simulink model "euler321_I2B_12B_with_contracts_EUL001_PP"  (R2017b)
settings: Solver=FixedStepDiscrete  StartTime=0.0  StopTime=10.0  FixedStep=0.010000  RelTol=1e-3  EnableMultiTasking=on
model workspace (MAT data in the model file):
  ContractValidatorBlocksMap = containers.Map
  ContractValidatorBlocksMap.serialization.keys = {'euler321_I2B_12B_with_contracts/euler321_I2B_12B_euler321_Spec/validator', 'euler321_I2B_12B_with_contracts_EUL001/euler321_I2B_12B_euler321_Spec/validator'}
  ContractValidatorBlocksMap.serialization.values{1}.block = 'euler321_I2B_12B_with_contracts/euler321_I2B_12B_euler321_Spec/validator'
  ContractValidatorBlocksMap.serialization.values{1}.assumePorts = 0
  ContractValidatorBlocksMap.serialization.values{1}.guaranteePorts = 9
  ContractValidatorBlocksMap.serialization.values{1}.modeBlocksPorts = 0
  ContractValidatorBlocksMap.serialization.values{1}.portHandles.Inport = [1936.00256348 1938.00256348 1940.00256348 1942.00256348 1944.00256348 1946.00256348 1948.00158691 1950.00256348 1952.00256348]
  ContractValidatorBlocksMap.serialization.values{1}.portHandles.Outport = 2039.00244141
  ContractValidatorBlocksMap.serialization.values{1}.portHandles.Enable = []
  ContractValidatorBlocksMap.serialization.values{1}.portHandles.Trigger = []
  ContractValidatorBlocksMap.serialization.values{1}.portHandles.State = []
  ContractValidatorBlocksMap.serialization.values{1}.portHandles.LConn = []
  ContractValidatorBlocksMap.serialization.values{1}.portHandles.RConn = []
  ContractValidatorBlocksMap.serialization.values{1}.portHandles.Ifaction = []
  ContractValidatorBlocksMap.serialization.values{1}.portHandles.Reset = []
  ContractValidatorBlocksMap.serialization.values{1}.portConnectivity(1).Type = '1'
  ContractValidatorBlocksMap.serialization.values{1}.portConnectivity(1).Position = [2610 2845]
  ContractValidatorBlocksMap.serialization.values{1}.portConnectivity(1).SrcBlock = 1300.00341797
  ContractValidatorBlocksMap.serialization.values{1}.portConnectivity(1).SrcPort = 0
  ContractValidatorBlocksMap.serialization.values{1}.portConnectivity(1).DstBlock = []
  ContractValidatorBlocksMap.serialization.values{1}.portConnectivity(1).DstPort = []
  ContractValidatorBlocksMap.serialization.values{1}.portConnectivity(2).Type = '2'
  ContractValidatorBlocksMap.serialization.values{1}.portConnectivity(2).Position = [2610 2885]
  ContractValidatorBlocksMap.serialization.values{1}.portConnectivity(2).SrcBlock = 1307.00341797
  ContractValidatorBlocksMap.serialization.values{1}.portConnectivity(2).SrcPort = 0
  ContractValidatorBlocksMap.serialization.values{1}.portConnectivity(2).DstBlock = []
  ContractValidatorBlocksMap.serialization.values{1}.portConnectivity(2).DstPort = []
  ContractValidatorBlocksMap.serialization.values{1}.portConnectivity(3).Type = '3'
  ContractValidatorBlocksMap.serialization.values{1}.portConnectivity(3).Position = [2610 2925]
  ContractValidatorBlocksMap.serialization.values{1}.portConnectivity(3).SrcBlock = 1314.00280762
  ContractValidatorBlocksMap.serialization.values{1}.portConnectivity(3).SrcPort = 0
  ContractValidatorBlocksMap.serialization.values{1}.portConnectivity(3).DstBlock = []
  ContractValidatorBlocksMap.serialization.values{1}.portConnectivity(3).DstPort = []
  ContractValidatorBlocksMap.serialization.values{1}.portConnectivity(4).Type = '4'
  ContractValidatorBlocksMap.serialization.values{1}.portConnectivity(4).Position = [2610 2965]
  ContractValidatorBlocksMap.serialization.values{1}.portConnectivity(4).SrcBlock = 1318.00280762
  ContractValidatorBlocksMap.serialization.values{1}.portConnectivity(4).SrcPort = 0
  ContractValidatorBlocksMap.serialization.values{1}.portConnectivity(4).DstBlock = []
  ContractValidatorBlocksMap.serialization.values{1}.portConnectivity(4).DstPort = []
  ContractValidatorBlocksMap.serialization.values{1}.portConnectivity(5).Type = '5'
  ContractValidatorBlocksMap.serialization.values{1}.portConnectivity(5).Position = [2610 3005]
  ContractValidatorBlocksMap.serialization.values{1}.portConnectivity(5).SrcBlock = 1326.00292969
  ContractValidatorBlocksMap.serialization.values{1}.portConnectivity(5).SrcPort = 0
  ContractValidatorBlocksMap.serialization.values{1}.portConnectivity(5).DstBlock = []
  ContractValidatorBlocksMap.serialization.values{1}.portConnectivity(5).DstPort = []
  ContractValidatorBlocksMap.serialization.values{1}.portConnectivity(6).Type = '6'
  ContractValidatorBlocksMap.serialization.values{1}.portConnectivity(6).Position = [2610 3045]
  ContractValidatorBlocksMap.serialization.values{1}.portConnectivity(6).SrcBlock = 1330.00341797
  ContractValidatorBlocksMap.serialization.values{1}.portConnectivity(6).SrcPort = 0
  ContractValidatorBlocksMap.serialization.values{1}.portConnectivity(6).DstBlock = []
  ContractValidatorBlocksMap.serialization.values{1}.portConnectivity(6).DstPort = []
  ContractValidatorBlocksMap.serialization.values{1}.portConnectivity(7).Type = '7'
  ContractValidatorBlocksMap.serialization.values{1}.portConnectivity(7).Position = [2610 3085]
  ContractValidatorBlocksMap.serialization.values{1}.portConnectivity(7).SrcBlock = 1337.00341797
  ContractValidatorBlocksMap.serialization.values{1}.portConnectivity(7).SrcPort = 0
  ContractValidatorBlocksMap.serialization.values{1}.portConnectivity(7).DstBlock = []
  ContractValidatorBlocksMap.serialization.values{1}.portConnectivity(7).DstPort = []
  ContractValidatorBlocksMap.serialization.values{1}.portConnectivity(8).Type = '8'
  ContractValidatorBlocksMap.serialization.values{1}.portConnectivity(8).Position = [2610 3125]
  ContractValidatorBlocksMap.serialization.values{1}.portConnectivity(8).SrcBlock = 1341.00341797
  ContractValidatorBlocksMap.serialization.values{1}.portConnectivity(8).SrcPort = 0
  ContractValidatorBlocksMap.serialization.values{1}.portConnectivity(8).DstBlock = []
  ContractValidatorBlocksMap.serialization.values{1}.portConnectivity(8).DstPort = []
  ContractValidatorBlocksMap.serialization.values{1}.portConnectivity(9).Type = '9'
  ContractValidatorBlocksMap.serialization.values{1}.portConnectivity(9).Position = [2610 3165]
  ContractValidatorBlocksMap.serialization.values{1}.portConnectivity(9).SrcBlock = 1348.00476074
  ContractValidatorBlocksMap.serialization.values{1}.portConnectivity(9).SrcPort = 0
  ContractValidatorBlocksMap.serialization.values{1}.portConnectivity(9).DstBlock = []
  ContractValidatorBlocksMap.serialization.values{1}.portConnectivity(9).DstPort = []
  ContractValidatorBlocksMap.serialization.values{1}.portConnectivity(10).Type = '1'
  ContractValidatorBlocksMap.serialization.values{1}.portConnectivity(10).Position = [2650 3005]
  ContractValidatorBlocksMap.serialization.values{1}.portConnectivity(10).SrcBlock = []
  ContractValidatorBlocksMap.serialization.values{1}.portConnectivity(10).SrcPort = []
  ContractValidatorBlocksMap.serialization.values{1}.portConnectivity(10).DstBlock = 1447.00341797
  ContractValidatorBlocksMap.serialization.values{1}.portConnectivity(10).DstPort = 0
  ContractValidatorBlocksMap.serialization.values{2}.block = 'euler321_I2B_12B_with_contracts_EUL001/euler321_I2B_12B_euler321_Spec/validator'
  ContractValidatorBlocksMap.serialization.values{2}.assumePorts = 0
  ContractValidatorBlocksMap.serialization.values{2}.guaranteePorts = 9
  ContractValidatorBlocksMap.serialization.values{2}.modeBlocksPorts = 0
  ContractValidatorBlocksMap.serialization.values{2}.portHandles.Inport = [497.151367188 498.151367188 499.150512695 500.149414062 501.150268555 502.149169922 503.149047852 504.149536133 505.150024414]
  ContractValidatorBlocksMap.serialization.values{2}.portHandles.Outport = 506.149047852
  ContractValidatorBlocksMap.serialization.values{2}.portHandles.Enable = []
  ContractValidatorBlocksMap.serialization.values{2}.portHandles.Trigger = []
  ContractValidatorBlocksMap.serialization.values{2}.portHandles.State = []
  ContractValidatorBlocksMap.serialization.values{2}.portHandles.LConn = []
  ContractValidatorBlocksMap.serialization.values{2}.portHandles.RConn = []
  ContractValidatorBlocksMap.serialization.values{2}.portHandles.Ifaction = []
  ContractValidatorBlocksMap.serialization.values{2}.portHandles.Reset = []
  ContractValidatorBlocksMap.serialization.values{2}.portConnectivity(1).Type = '1'
  ContractValidatorBlocksMap.serialization.values{2}.portConnectivity(1).Position = [2610 2845]
  ContractValidatorBlocksMap.serialization.values{2}.portConnectivity(1).SrcBlock = 243.150024414
  ContractValidatorBlocksMap.serialization.values{2}.portConnectivity(1).SrcPort = 0
  ContractValidatorBlocksMap.serialization.values{2}.portConnectivity(1).DstBlock = []
  ContractValidatorBlocksMap.serialization.values{2}.portConnectivity(1).DstPort = []
  ContractValidatorBlocksMap.serialization.values{2}.portConnectivity(2).Type = '2'
  ContractValidatorBlocksMap.serialization.values{2}.portConnectivity(2).Position = [2610 2885]
  ContractValidatorBlocksMap.serialization.values{2}.portConnectivity(2).SrcBlock = 247.150024414
  ContractValidatorBlocksMap.serialization.values{2}.portConnectivity(2).SrcPort = 0
  ContractValidatorBlocksMap.serialization.values{2}.portConnectivity(2).DstBlock = []
  ContractValidatorBlocksMap.serialization.values{2}.portConnectivity(2).DstPort = []
  ContractValidatorBlocksMap.serialization.values{2}.portConnectivity(3).Type = '3'
  ContractValidatorBlocksMap.serialization.values{2}.portConnectivity(3).Position = [2610 2925]
  ContractValidatorBlocksMap.serialization.values{2}.portConnectivity(3).SrcBlock = 251.153320312
  ContractValidatorBlocksMap.serialization.values{2}.portConnectivity(3).SrcPort = 0
  ContractValidatorBlocksMap.serialization.values{2}.portConnectivity(3).DstBlock = []
  ContractValidatorBlocksMap.serialization.values{2}.portConnectivity(3).DstPort = []
  ContractValidatorBlocksMap.serialization.values{2}.portConnectivity(4).Type = '4'
  ContractValidatorBlocksMap.serialization.values{2}.portConnectivity(4).Position = [2610 2965]
  ContractValidatorBlocksMap.serialization.values{2}.portConnectivity(4).SrcBlock = 255.153564453
  ContractValidatorBlocksMap.serialization.values{2}.portConnectivity(4).SrcPort = 0
  ContractValidatorBlocksMap.serialization.values{2}.portConnectivity(4).DstBlock = []
  ContractValidatorBlocksMap.serialization.values{2}.portConnectivity(4).DstPort = []
  ContractValidatorBlocksMap.serialization.values{2}.portConnectivity(5).Type = '5'
  ContractValidatorBlocksMap.serialization.values{2}.portConnectivity(5).Position = [2610 3005]
  ContractValidatorBlocksMap.serialization.values{2}.portConnectivity(5).SrcBlock = 259.148925781
  ContractValidatorBlocksMap.serialization.values{2}.portConnectivity(5).SrcPort = 0
  ContractValidatorBlocksMap.serialization.values{2}.portConnectivity(5).DstBlock = []
  ContractValidatorBlocksMap.serialization.values{2}.portConnectivity(5).DstPort = []
  ContractValidatorBlocksMap.serialization.values{2}.portConnectivity(6).Type = '6'
  ContractValidatorBlocksMap.serialization.values{2}.portConnectivity(6).Position = [2610 3045]
  ContractValidatorBlocksMap.serialization.values{2}.portConnectivity(6).SrcBlock = 263.154296875
  ContractValidatorBlocksMap.serialization.values{2}.portConnectivity(6).SrcPort = 0
  ContractValidatorBlocksMap.serialization.values{2}.portConnectivity(6).DstBlock = []
  ContractValidatorBlocksMap.serialization.values{2}.portConnectivity(6).DstPort = []
  ContractValidatorBlocksMap.serialization.values{2}.portConnectivity(7).Type = '7'
  ContractValidatorBlocksMap.serialization.values{2}.portConnectivity(7).Position = [2610 3085]
  ContractValidatorBlocksMap.serialization.values{2}.portConnectivity(7).SrcBlock = 267.154418945
  ContractValidatorBlocksMap.serialization.values{2}.portConnectivity(7).SrcPort = 0
  ContractValidatorBlocksMap.serialization.values{2}.portConnectivity(7).DstBlock = []
  ContractValidatorBlocksMap.serialization.values{2}.portConnectivity(7).DstPort = []
  ContractValidatorBlocksMap.serialization.values{2}.portConnectivity(8).Type = '8'
  ContractValidatorBlocksMap.serialization.values{2}.portConnectivity(8).Position = [2610 3125]
  ContractValidatorBlocksMap.serialization.values{2}.portConnectivity(8).SrcBlock = 271.148925781
  ContractValidatorBlocksMap.serialization.values{2}.portConnectivity(8).SrcPort = 0
  ContractValidatorBlocksMap.serialization.values{2}.portConnectivity(8).DstBlock = []
  ContractValidatorBlocksMap.serialization.values{2}.portConnectivity(8).DstPort = []
  ContractValidatorBlocksMap.serialization.values{2}.portConnectivity(9).Type = '9'
  ContractValidatorBlocksMap.serialization.values{2}.portConnectivity(9).Position = [2610 3165]
  ContractValidatorBlocksMap.serialization.values{2}.portConnectivity(9).SrcBlock = 275.153442383
  ContractValidatorBlocksMap.serialization.values{2}.portConnectivity(9).SrcPort = 0
  ContractValidatorBlocksMap.serialization.values{2}.portConnectivity(9).DstBlock = []
  ContractValidatorBlocksMap.serialization.values{2}.portConnectivity(9).DstPort = []
  ContractValidatorBlocksMap.serialization.values{2}.portConnectivity(10).Type = '1'
  ContractValidatorBlocksMap.serialization.values{2}.portConnectivity(10).Position = [2650 3005]
  ContractValidatorBlocksMap.serialization.values{2}.portConnectivity(10).SrcBlock = []
  ContractValidatorBlocksMap.serialization.values{2}.portConnectivity(10).SrcPort = []
  ContractValidatorBlocksMap.serialization.values{2}.portConnectivity(10).DstBlock = 342.152099609
  ContractValidatorBlocksMap.serialization.values{2}.portConnectivity(10).DstPort = 0
  ContractValidatorBlocksMap.serialization.uniformity = 0
  ContractValidatorBlocksMap.serialization.keyType = 'char'
  ContractValidatorBlocksMap.serialization.valueType = 'any'
  already_pp = 1
  compositionalMap.analysisNames = {'euler321_I2B_12B_with_contracts_EUL001_PP/COORDINATETRANSFORM_newline_EULER321_newline__lpar_INERTIALTOBODY_rpar_'}
  compositionalMap.compositionalOptions = {{''}}
  compositionalMap.selectedOptions = 1
  maskControlsMap = containers.Map
  maskControlsMap.serialization.keys = {'euler321_I2B_12B_with_contracts_EUL001_PP/euler321_I2B_12B_euler321_Spec/EUL001_1', 'euler321_I2B_12B_with_contracts_EUL001_PP/euler321_I2B_12B_euler321_Spec/EUL001_2', 'euler321_I2B_12B_with_contracts_EUL001_PP/euler321_I2B_12B_euler321_Spec/EUL001_3', 'euler321_I2B_12B_with_contracts_EUL001_PP/euler321_I2B_12B_euler321_Spec/EUL001_4', 'euler321_I2B_12B_with_contracts_EUL001_PP/euler321_I2B_12B_euler321_Spec/EUL001_5', 'euler321_I2B_12B_with_contracts_EUL001_PP/euler321_I2B_12B_euler321_Spec/EUL001_6', 'euler321_I2B_12B_with_contracts_EUL001_PP/euler321_I2B_12B_euler321_Spec/EUL001_7', 'euler321_I2B_12B_with_contracts_EUL001_PP/euler321_I2B_12B_euler321_Spec/EUL001_8', 'euler321_I2B_12B_with_contracts_EUL001_PP/euler321_I2B_12B_euler321_Spec/EUL001_9'}
  maskControlsMap.serialization.values = {{'Display_counter_example_as_signals', 'Display_counter_example_as_tables', 'Display_counter_example_as_HTML_tables', 'Generate_an_outer_model_for_the_counter_example', 'Generate_an_inner_model_for_the_counter_example'}, {'Display_counter_example_as_signals', 'Display_counter_example_as_tables', 'Display_counter_example_as_HTML_tables', 'Generate_an_outer_model_for_the_counter_example', 'Generate_an_inner_model_for_the_counter_example'}, {'Display_counter_example_as_signals', 'Display_counter_example_as_tables', 'Display_counter_example_as_HTML_tables', 'Generate_an_outer_model_for_the_counter_example', 'Generate_an_inner_model_for_the_counter_example'}, {'Display_counter_example_as_signals', 'Display_counter_example_as_tables', 'Display_counter_example_as_HTML_tables', 'Generate_an_outer_model_for_the_counter_example', 'Generate_an_inner_model_for_the_counter_example'}, {'Display_counter_example_as_signals', 'Display_counter_example_as_tables', 'Display_counter_example_as_HTML_tables', 'Generate_an_outer_model_for_the_counter_example', 'Generate_an_inner_model_for_the_counter_example'}, {'Display_counter_example_as_signals', 'Display_counter_example_as_tables', 'Display_counter_example_as_HTML_tables', 'Generate_an_outer_model_for_the_counter_example', 'Generate_an_inner_model_for_the_counter_example'}, {'Display_counter_example_as_signals', 'Display_counter_example_as_tables', 'Display_counter_example_as_HTML_tables', 'Generate_an_outer_model_for_the_counter_example', 'Generate_an_inner_model_for_the_counter_example'}, {'Display_counter_example_as_signals', 'Display_counter_example_as_tables', 'Display_counter_example_as_HTML_tables', 'Generate_an_outer_model_for_the_counter_example', 'Generate_an_inner_model_for_the_counter_example'}, {'Display_counter_example_as_signals', 'Display_counter_example_as_tables', 'Display_counter_example_as_HTML_tables', 'Generate_an_outer_model_for_the_counter_example', 'Generate_an_inner_model_for_the_counter_example'}}
  maskControlsMap.serialization.uniformity = 0
  maskControlsMap.serialization.keyType = 'char'
  maskControlsMap.serialization.valueType = 'any'
  nodeNameToBlockNameMap : containers.Map (value not decoded)
  verificationResults : struct (value not decoded)
undefined symbols (not defined in the file): contractAfterSimulation, contractBeforeSimulation, ContractBlock, ContractGuaranteeBlock, ContractValidatorBlock, saveValidatorParameters
settings Model: Creator=elliocm  LastModifiedBy=hbourbou
settings DataIOCC: LimitDataPoints=on  SaveFormat=StructureWithTime  SignalLoggingSaveFormat=ModelDataLogs
settings OptimizationCC: ExpressionDepthLimit=2147483647  LifeSpan=inf
settings DebuggingCC: AlgebraicLoopMsg=error  ArtificialAlgebraicLoopMsg=error  UnderspecifiedInitializationDetection=Classic  MergeDetectMultiDrivingBlocksExec=none  SolverPrmCheckMsg=warning  SingleTaskRateTransMsg=error  FcnCallInpInsideContextMsg=warning  StateNameClashWarn=warning  SFUnexpectedBacktrackingDiag=warning  SFNoUnconditionalDefaultTransitionDiag=warning  SFExecutionAtInitializationDiag=none
settings HardwareCC: ProdBitPerPointer=32  ProdBitPerSizeT=32  ProdBitPerPtrDiffT=32  ProdLargestAtomicFloat=None  ProdIntDivRoundTo=Undefined  ProdEndianess=Unspecified  ProdWordSize=32  ProdHWDeviceType=32-bit Generic
settings ModelReferenceCC: PropagateSignalLabelsOutOfModel=off
settings CodeAppCC: StateflowObjectComments=on
settings GRTTargetCC: TargetLangStandard=C89/C90 (ANSI)  GeneratePreprocessorConditionals=Disable all  CombineOutputUpdateFcns=off  GRTInterface=on
settings ConfigComp: CovMetricSettings=dw  CovHtmlReporting=on  CovSaveCumulativeToWorkspaceVar=on  CovSaveSingleToWorkspaceVar=on  CovExternalEMLEnable=off

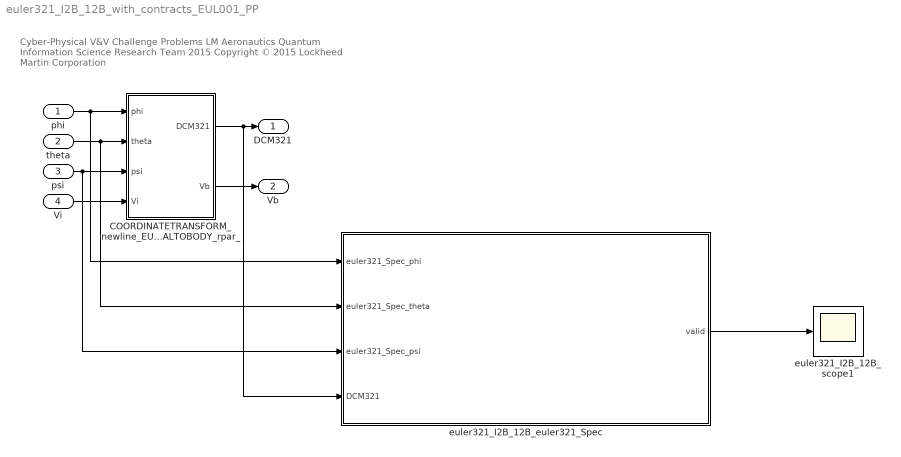
== system euler321_I2B_12B_with_contracts_EUL001_PP ==
  note: Cyber-Physical V&V Challenge Problems
      | LM Aeronautics Quantum Information Science Research Team 2015
      | Copyright © 2015 Lockheed Martin Corporation
  phi : Inport  OutDataTypeStr=double
  theta : Inport  Port=2  OutDataTypeStr=double
  psi : Inport  Port=3  OutDataTypeStr=double
  Vi : Inport  Port=4  OutDataTypeStr=double  PortDimensions=3
  COORDINATETRANSFORM_newline_EULER321_newline__lpar_INERTIALTOBODY_rpar_ : Subsystem  TreatAsAtomicUnit=on
  euler321_I2B_12B_euler321_Spec : Subsystem  TreatAsAtomicUnit=on  mask(ContractBlock){ContractBlockType=ContractBlock}
      mask init:
      | set_param(gcb, 'LinkStatus', 'none');
      mask DialogControl DescTextVar Prompt: Contract block
      mask Display:
      | text(0.5, 0.5, '{\bf\fontsize{20}Contract}', 'hor', 'center', 'texmode','on');
      | blocks = find_system(gcb, 'LookUnderMasks','all', 'SearchDepth',1,'BlockType','Inport');
      | for i = 1 : length(blocks)
      |     blockName = get_param(blocks(i), 'Name');
      |     [path, blockName] = fileparts(char(blockName));
      |     port_label('input', i, blockName);
      | end
      | 
      | blocks = find_system(gcb, 'LookUnderMasks','all', 'SearchDepth',1,'BlockType','Outport');
      | for i = 1 : length(blocks)
      |     blockName = get_param(blocks(i), 'Name');
      |     [path, blockName] = fileparts(char(blockName));
      |     port_label('output', i, blockName);
      | end
  euler321_I2B_12B_scope1 : Scope
  DCM321 : Outport  VectorParamsAs1DForOutWhenUnconnected=off
  Vb : Outport  Port=2  VectorParamsAs1DForOutWhenUnconnected=off
  wires:
  COORDINATETRANSFORM_newline_EULER321_newline__lpar_INERTIALTOBODY_rpar_/1(DCM321) -> euler321_I2B_12B_euler321_Spec/4(DCM321), DCM321/1
  COORDINATETRANSFORM_newline_EULER321_newline__lpar_INERTIALTOBODY_rpar_/2(Vb) -> Vb/1
  phi/1 -> COORDINATETRANSFORM_newline_EULER321_newline__lpar_INERTIALTOBODY_rpar_/1(phi), euler321_I2B_12B_euler321_Spec/1(euler321_Spec_phi)
  theta/1 -> euler321_I2B_12B_euler321_Spec/2(euler321_Spec_theta), COORDINATETRANSFORM_newline_EULER321_newline__lpar_INERTIALTOBODY_rpar_/2(theta)
  psi/1 -> COORDINATETRANSFORM_newline_EULER321_newline__lpar_INERTIALTOBODY_rpar_/3(psi), euler321_I2B_12B_euler321_Spec/3(euler321_Spec_psi)
  Vi/1 -> COORDINATETRANSFORM_newline_EULER321_newline__lpar_INERTIALTOBODY_rpar_/4(Vi)
  euler321_I2B_12B_euler321_Spec/1(valid) -> euler321_I2B_12B_scope1/1

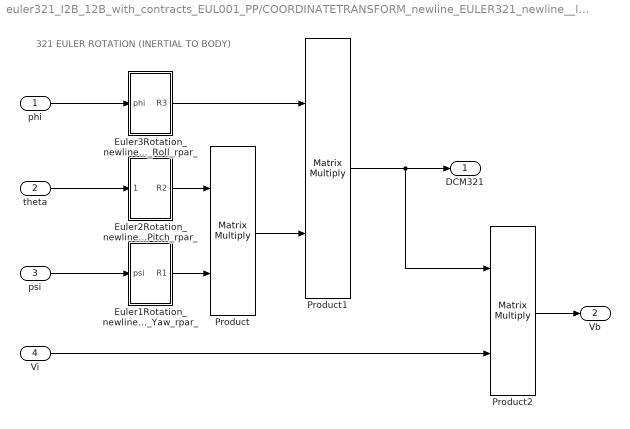
== system euler321_I2B_12B_with_contracts_EUL001_PP/COORDINATETRANSFORM_newline_EULER321_newline__lpar_INERTIALTOBODY_rpar_ ==
  note: 321 EULER ROTATION (INERTIAL TO BODY)
  phi : Inport
  theta : Inport  Port=2
  psi : Inport  Port=3
  Vi : Inport  Port=4
  Euler1Rotation_newline__lpar_Yaw_rpar_ : Subsystem  TreatAsAtomicUnit=on
  Euler2Rotation_newline__lpar_Pitch_rpar_ : Subsystem  TreatAsAtomicUnit=on
  Euler3Rotation_newline__lpar_Roll_rpar_ : Subsystem  TreatAsAtomicUnit=on
  Product : Product  Multiplication=Matrix(*)  RndMeth=Zero
  Product1 : Product  Multiplication=Matrix(*)  RndMeth=Zero
  Product2 : Product  Multiplication=Matrix(*)  RndMeth=Zero
  DCM321 : Outport  VectorParamsAs1DForOutWhenUnconnected=off
  Vb : Outport  Port=2  VectorParamsAs1DForOutWhenUnconnected=off
  wires:
  Euler2Rotation_newline__lpar_Pitch_rpar_/1(R2) -> Product/1
  Euler1Rotation_newline__lpar_Yaw_rpar_/1(R1) -> Product/2
  Euler3Rotation_newline__lpar_Roll_rpar_/1(R3) -> Product1/1
  Product/1 -> Product1/2
  Product1/1 -> DCM321/1, Product2/1
  Product2/1 -> Vb/1
  phi/1 -> Euler3Rotation_newline__lpar_Roll_rpar_/1(phi)
  theta/1 -> Euler2Rotation_newline__lpar_Pitch_rpar_/1(theta)
  psi/1 -> Euler1Rotation_newline__lpar_Yaw_rpar_/1(psi)
  Vi/1 -> Product2/2

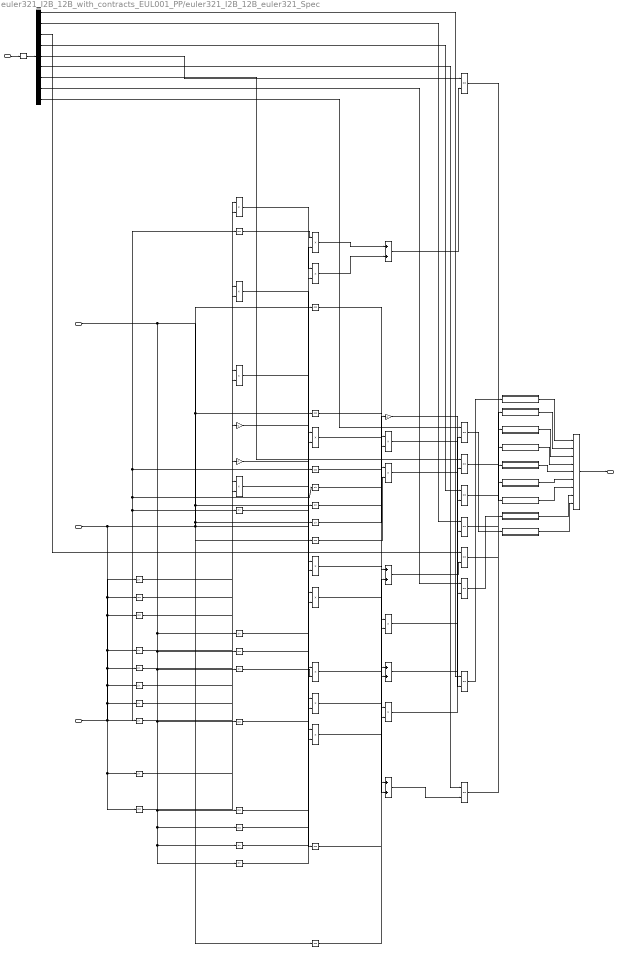
== system euler321_I2B_12B_with_contracts_EUL001_PP/euler321_I2B_12B_euler321_Spec ==
  euler321_Spec_phi : Inport  OutDataTypeStr=double
  euler321_Spec_theta : Inport  Port=2  OutDataTypeStr=double
  euler321_Spec_psi : Inport  Port=3  OutDataTypeStr=double
  DCM321 : Inport  Port=4
  Demux3 : Demux  Outputs=9
  EUL001_1 : Subsystem  TreatAsAtomicUnit=on  mask(ContractGuaranteeBlock){ContractBlockType=ContractGuaranteeBlock}
      mask init:
      | set_param(gcb, 'LinkStatus', 'none');
      mask DialogControl DescTextVar Prompt: Guarantee block
      mask DialogControl Display_counter_example_as_signals Prompt: Display counter example as signals
      mask DialogControl Display_counter_example_as_signals Callback: displayCexSignals(1, 3);
      mask DialogControl Display_counter_example_as_tables Prompt: Display counter example as tables
      mask DialogControl Display_counter_example_as_tables Callback: displayCexTables(1, 3);
      mask DialogControl Display_counter_example_as_HTML_tables Prompt: Display counter example as HTML tables
      mask DialogControl Display_counter_example_as_HTML_tables Callback: displayCexHtmlTables(1, 3);
      mask DialogControl Generate_an_outer_model_for_the_counter_example Prompt: Generate an outer model for the counter example
      mask DialogControl Generate_an_outer_model_for_the_counter_example Callback: generateModelWithSignalBuilders(1, 3, 2);
      mask DialogControl Generate_an_inner_model_for_the_counter_example Prompt: Generate an inner model for the counter example
      mask DialogControl Generate_an_inner_model_for_the_counter_example Callback: generateModelWithSignalBuilders(1, 3, 1);
  EUL001_2 : Subsystem  TreatAsAtomicUnit=on  mask(ContractGuaranteeBlock){ContractBlockType=ContractGuaranteeBlock}
      mask init:
      | set_param(gcb, 'LinkStatus', 'none');
      mask DialogControl DescTextVar Prompt: Guarantee block
      mask DialogControl Display_counter_example_as_signals Prompt: Display counter example as signals
      mask DialogControl Display_counter_example_as_signals Callback: displayCexSignals(1, 4);
      mask DialogControl Display_counter_example_as_tables Prompt: Display counter example as tables
      mask DialogControl Display_counter_example_as_tables Callback: displayCexTables(1, 4);
      mask DialogControl Display_counter_example_as_HTML_tables Prompt: Display counter example as HTML tables
      mask DialogControl Display_counter_example_as_HTML_tables Callback: displayCexHtmlTables(1, 4);
      mask DialogControl Generate_an_outer_model_for_the_counter_example Prompt: Generate an outer model for the counter example
      mask DialogControl Generate_an_outer_model_for_the_counter_example Callback: generateModelWithSignalBuilders(1, 4, 2);
      mask DialogControl Generate_an_inner_model_for_the_counter_example Prompt: Generate an inner model for the counter example
      mask DialogControl Generate_an_inner_model_for_the_counter_example Callback: generateModelWithSignalBuilders(1, 4, 1);
  EUL001_3 : Subsystem  TreatAsAtomicUnit=on  mask(ContractGuaranteeBlock){ContractBlockType=ContractGuaranteeBlock}
      mask init:
      | set_param(gcb, 'LinkStatus', 'none');
      mask DialogControl DescTextVar Prompt: Guarantee block
      mask DialogControl Display_counter_example_as_signals Prompt: Display counter example as signals
      mask DialogControl Display_counter_example_as_signals Callback: displayCexSignals(1, 5);
      mask DialogControl Display_counter_example_as_tables Prompt: Display counter example as tables
      mask DialogControl Display_counter_example_as_tables Callback: displayCexTables(1, 5);
      mask DialogControl Display_counter_example_as_HTML_tables Prompt: Display counter example as HTML tables
      mask DialogControl Display_counter_example_as_HTML_tables Callback: displayCexHtmlTables(1, 5);
      mask DialogControl Generate_an_outer_model_for_the_counter_example Prompt: Generate an outer model for the counter example
      mask DialogControl Generate_an_outer_model_for_the_counter_example Callback: generateModelWithSignalBuilders(1, 5, 2);
      mask DialogControl Generate_an_inner_model_for_the_counter_example Prompt: Generate an inner model for the counter example
      mask DialogControl Generate_an_inner_model_for_the_counter_example Callback: generateModelWithSignalBuilders(1, 5, 1);
  EUL001_4 : Subsystem  TreatAsAtomicUnit=on  mask(ContractGuaranteeBlock){ContractBlockType=ContractGuaranteeBlock}
      mask init:
      | set_param(gcb, 'LinkStatus', 'none');
      mask DialogControl DescTextVar Prompt: Guarantee block
      mask DialogControl Display_counter_example_as_signals Prompt: Display counter example as signals
      mask DialogControl Display_counter_example_as_signals Callback: displayCexSignals(1, 6);
      mask DialogControl Display_counter_example_as_tables Prompt: Display counter example as tables
      mask DialogControl Display_counter_example_as_tables Callback: displayCexTables(1, 6);
      mask DialogControl Display_counter_example_as_HTML_tables Prompt: Display counter example as HTML tables
      mask DialogControl Display_counter_example_as_HTML_tables Callback: displayCexHtmlTables(1, 6);
      mask DialogControl Generate_an_outer_model_for_the_counter_example Prompt: Generate an outer model for the counter example
      mask DialogControl Generate_an_outer_model_for_the_counter_example Callback: generateModelWithSignalBuilders(1, 6, 2);
      mask DialogControl Generate_an_inner_model_for_the_counter_example Prompt: Generate an inner model for the counter example
      mask DialogControl Generate_an_inner_model_for_the_counter_example Callback: generateModelWithSignalBuilders(1, 6, 1);
  EUL001_5 : Subsystem  TreatAsAtomicUnit=on  mask(ContractGuaranteeBlock){ContractBlockType=ContractGuaranteeBlock}
      mask init:
      | set_param(gcb, 'LinkStatus', 'none');
      mask DialogControl DescTextVar Prompt: Guarantee block
      mask DialogControl Display_counter_example_as_signals Prompt: Display counter example as signals
      mask DialogControl Display_counter_example_as_signals Callback: displayCexSignals(1, 7);
      mask DialogControl Display_counter_example_as_tables Prompt: Display counter example as tables
      mask DialogControl Display_counter_example_as_tables Callback: displayCexTables(1, 7);
      mask DialogControl Display_counter_example_as_HTML_tables Prompt: Display counter example as HTML tables
      mask DialogControl Display_counter_example_as_HTML_tables Callback: displayCexHtmlTables(1, 7);
      mask DialogControl Generate_an_outer_model_for_the_counter_example Prompt: Generate an outer model for the counter example
      mask DialogControl Generate_an_outer_model_for_the_counter_example Callback: generateModelWithSignalBuilders(1, 7, 2);
      mask DialogControl Generate_an_inner_model_for_the_counter_example Prompt: Generate an inner model for the counter example
      mask DialogControl Generate_an_inner_model_for_the_counter_example Callback: generateModelWithSignalBuilders(1, 7, 1);
  EUL001_6 : Subsystem  TreatAsAtomicUnit=on  mask(ContractGuaranteeBlock){ContractBlockType=ContractGuaranteeBlock}
      mask init:
      | set_param(gcb, 'LinkStatus', 'none');
      mask DialogControl DescTextVar Prompt: Guarantee block
      mask DialogControl Display_counter_example_as_signals Prompt: Display counter example as signals
      mask DialogControl Display_counter_example_as_signals Callback: displayCexSignals(1, 8);
      mask DialogControl Display_counter_example_as_tables Prompt: Display counter example as tables
      mask DialogControl Display_counter_example_as_tables Callback: displayCexTables(1, 8);
      mask DialogControl Display_counter_example_as_HTML_tables Prompt: Display counter example as HTML tables
      mask DialogControl Display_counter_example_as_HTML_tables Callback: displayCexHtmlTables(1, 8);
      mask DialogControl Generate_an_outer_model_for_the_counter_example Prompt: Generate an outer model for the counter example
      mask DialogControl Generate_an_outer_model_for_the_counter_example Callback: generateModelWithSignalBuilders(1, 8, 2);
      mask DialogControl Generate_an_inner_model_for_the_counter_example Prompt: Generate an inner model for the counter example
      mask DialogControl Generate_an_inner_model_for_the_counter_example Callback: generateModelWithSignalBuilders(1, 8, 1);
  EUL001_7 : Subsystem  TreatAsAtomicUnit=on  mask(ContractGuaranteeBlock){ContractBlockType=ContractGuaranteeBlock}
      mask init:
      | set_param(gcb, 'LinkStatus', 'none');
      mask DialogControl DescTextVar Prompt: Guarantee block
      mask DialogControl Display_counter_example_as_signals Prompt: Display counter example as signals
      mask DialogControl Display_counter_example_as_signals Callback: displayCexSignals(1, 1);
      mask DialogControl Display_counter_example_as_tables Prompt: Display counter example as tables
      mask DialogControl Display_counter_example_as_tables Callback: displayCexTables(1, 1);
      mask DialogControl Display_counter_example_as_HTML_tables Prompt: Display counter example as HTML tables
      mask DialogControl Display_counter_example_as_HTML_tables Callback: displayCexHtmlTables(1, 1);
      mask DialogControl Generate_an_outer_model_for_the_counter_example Prompt: Generate an outer model for the counter example
      mask DialogControl Generate_an_outer_model_for_the_counter_example Callback: generateModelWithSignalBuilders(1, 1, 2);
      mask DialogControl Generate_an_inner_model_for_the_counter_example Prompt: Generate an inner model for the counter example
      mask DialogControl Generate_an_inner_model_for_the_counter_example Callback: generateModelWithSignalBuilders(1, 1, 1);
  EUL001_8 : Subsystem  TreatAsAtomicUnit=on  mask(ContractGuaranteeBlock){ContractBlockType=ContractGuaranteeBlock}
      mask init:
      | set_param(gcb, 'LinkStatus', 'none');
      mask DialogControl DescTextVar Prompt: Guarantee block
      mask DialogControl Display_counter_example_as_signals Prompt: Display counter example as signals
      mask DialogControl Display_counter_example_as_signals Callback: displayCexSignals(1, 2);
      mask DialogControl Display_counter_example_as_tables Prompt: Display counter example as tables
      mask DialogControl Display_counter_example_as_tables Callback: displayCexTables(1, 2);
      mask DialogControl Display_counter_example_as_HTML_tables Prompt: Display counter example as HTML tables
      mask DialogControl Display_counter_example_as_HTML_tables Callback: displayCexHtmlTables(1, 2);
      mask DialogControl Generate_an_outer_model_for_the_counter_example Prompt: Generate an outer model for the counter example
      mask DialogControl Generate_an_outer_model_for_the_counter_example Callback: generateModelWithSignalBuilders(1, 2, 2);
      mask DialogControl Generate_an_inner_model_for_the_counter_example Prompt: Generate an inner model for the counter example
      mask DialogControl Generate_an_inner_model_for_the_counter_example Callback: generateModelWithSignalBuilders(1, 2, 1);
  EUL001_9 : Subsystem  TreatAsAtomicUnit=on  mask(ContractGuaranteeBlock){ContractBlockType=ContractGuaranteeBlock}
      mask init:
      | set_param(gcb, 'LinkStatus', 'none');
      mask DialogControl DescTextVar Prompt: Guarantee block
      mask DialogControl Display_counter_example_as_signals Prompt: Display counter example as signals
      mask DialogControl Display_counter_example_as_signals Callback: displayCexSignals(1, 9);
      mask DialogControl Display_counter_example_as_tables Prompt: Display counter example as tables
      mask DialogControl Display_counter_example_as_tables Callback: displayCexTables(1, 9);
      mask DialogControl Display_counter_example_as_HTML_tables Prompt: Display counter example as HTML tables
      mask DialogControl Display_counter_example_as_HTML_tables Callback: displayCexHtmlTables(1, 9);
      mask DialogControl Generate_an_outer_model_for_the_counter_example Prompt: Generate an outer model for the counter example
      mask DialogControl Generate_an_outer_model_for_the_counter_example Callback: generateModelWithSignalBuilders(1, 9, 2);
      mask DialogControl Generate_an_inner_model_for_the_counter_example Prompt: Generate an inner model for the counter example
      mask DialogControl Generate_an_inner_model_for_the_counter_example Callback: generateModelWithSignalBuilders(1, 9, 1);
  Reshape : Reshape
  spec113_operator : RelationalOperator  Operator===  OutDataTypeStr=boolean  RndMeth=Simplest
  spec123_operator : RelationalOperator  Operator===  OutDataTypeStr=boolean  RndMeth=Simplest
  spec145_operator : RelationalOperator  Operator===  OutDataTypeStr=boolean  RndMeth=Simplest
  spec169_operator : RelationalOperator  Operator===  OutDataTypeStr=boolean  RndMeth=Simplest
  spec177_operator : RelationalOperator  Operator===  OutDataTypeStr=boolean  RndMeth=Simplest
  spec187_operator : RelationalOperator  Operator===  OutDataTypeStr=boolean  RndMeth=Simplest
  spec197_operator : RelationalOperator  Operator===  OutDataTypeStr=boolean  RndMeth=Simplest
  spec67_operator : RelationalOperator  Operator===  OutDataTypeStr=boolean  RndMeth=Simplest
  spec91_operator : RelationalOperator  Operator===  OutDataTypeStr=boolean  RndMeth=Simplest
  validator : M-S-Function  LoadFcn=saveValidatorParameters(gcb);  InitFcn=contractBeforeSimulation();  StopFcn=contractAfterSimulation();  FunctionName=contract  mask(ContractValidatorBlock){assumePorts=0, guaranteePorts=9, modePorts=0, ContractBlockType=ContractValidatorBlock, createInportsCheckbox=off}
      mask prompts: assumePorts "Assume ports     :"; guaranteePorts "Guarantee ports :"; modePorts "Mode ports        :"; createInportsCheckbox "Create inports and connect them automatically"
      mask init:
      | set_param(gcb,'LinkStatus','none');
      | contract_callback('inputs_callback',gcb);
      mask DialogControl DescTextVar Prompt: The validator block implements the following logic: <br> <br> <b>Sofar</b>(assume<sub>1</sub> <b>&#8743;</b> assume<sub>2</sub> <b>&#8743;</b> ... assume<sub>k</sub>) <b>&rarr;</b> (guarantee<sub>1</sub> <b>&#8743;</b> guarantee<sub>2</sub> <b>&#8743;</b> ... guarantee<sub>m</sub> <b>&#8743;</b>  mode<sub>1</sub> <b>&#8743;</b> mode<sub>2</sub> <b>&#8743;</b> ... <b>&#8743;</b> mode<sub>n</sub> )<br> where mode<sub>i</sub> = require<sub>i</sub> <b>&rarr;</b> ensure<sub>i</sub>
      mask Display:
      | color('black');
      | port_label('input',1,'guarantee');
      | port_label('input',2,'guarantee');
      | port_label('input',3,'guarantee');
      | port_label('input',4,'guarantee');
      | port_label('input',5,'guarantee');
      | port_label('input',6,'guarantee');
      | port_label('input',7,'guarantee');
      | port_label('input',8,'guarantee');
      | port_label('input',9,'guarantee');
      | port_label('output',1,'valid');
  xxeuler321_Spec_10_sin_call : Trigonometry
  xxeuler321_Spec_11_cos_call : Trigonometry  Operator=cos
  xxeuler321_Spec_12_operator : Product  OutDataTypeStr=double
  xxeuler321_Spec_13_operator : Product  OutDataTypeStr=double
  xxeuler321_Spec_14_cos_call : Trigonometry  Operator=cos
  xxeuler321_Spec_15_sin_call : Trigonometry
  xxeuler321_Spec_16_operator : Gain  Gain=-1  OutDataTypeStr=double
  xxeuler321_Spec_17_operator : Product  OutDataTypeStr=double
  xxeuler321_Spec_18_operator : Sum  OutDataTypeStr=double
  xxeuler321_Spec_19_sin_call : Trigonometry
  xxeuler321_Spec_1_cos_call : Trigonometry  Operator=cos
  xxeuler321_Spec_20_sin_call : Trigonometry
  xxeuler321_Spec_21_sin_call : Trigonometry
  xxeuler321_Spec_22_operator : Product  OutDataTypeStr=double
  xxeuler321_Spec_23_operator : Product  OutDataTypeStr=double
  xxeuler321_Spec_24_cos_call : Trigonometry  Operator=cos
  xxeuler321_Spec_25_cos_call : Trigonometry  Operator=cos
  xxeuler321_Spec_26_operator : Product  OutDataTypeStr=double
  xxeuler321_Spec_27_operator : Sum  OutDataTypeStr=double
  xxeuler321_Spec_28_sin_call : Trigonometry
  xxeuler321_Spec_29_cos_call : Trigonometry  Operator=cos
  xxeuler321_Spec_2_cos_call : Trigonometry  Operator=cos
  xxeuler321_Spec_30_operator : Product  OutDataTypeStr=double
  xxeuler321_Spec_31_cos_call : Trigonometry  Operator=cos
  xxeuler321_Spec_32_sin_call : Trigonometry
  xxeuler321_Spec_33_cos_call : Trigonometry  Operator=cos
  xxeuler321_Spec_34_operator : Product  OutDataTypeStr=double
  xxeuler321_Spec_35_operator : Product  OutDataTypeStr=double
  xxeuler321_Spec_36_sin_call : Trigonometry
  xxeuler321_Spec_37_sin_call : Trigonometry
  xxeuler321_Spec_38_operator : Product  OutDataTypeStr=double
  xxeuler321_Spec_39_operator : Sum  OutDataTypeStr=double
  xxeuler321_Spec_3_operator : Product  OutDataTypeStr=double
  xxeuler321_Spec_40_cos_call : Trigonometry  Operator=cos
  xxeuler321_Spec_41_sin_call : Trigonometry
  xxeuler321_Spec_42_sin_call : Trigonometry
  xxeuler321_Spec_43_operator : Product  OutDataTypeStr=double
  xxeuler321_Spec_44_operator : Product  OutDataTypeStr=double
  xxeuler321_Spec_45_sin_call : Trigonometry
  xxeuler321_Spec_46_cos_call : Trigonometry  Operator=cos
  xxeuler321_Spec_47_operator : Gain  Gain=-1  OutDataTypeStr=double
  xxeuler321_Spec_48_operator : Product  OutDataTypeStr=double
  xxeuler321_Spec_49_operator : Sum  OutDataTypeStr=double
  xxeuler321_Spec_4_cos_call : Trigonometry  Operator=cos
  xxeuler321_Spec_50_cos_call : Trigonometry  Operator=cos
  xxeuler321_Spec_51_cos_call : Trigonometry  Operator=cos
  xxeuler321_Spec_52_operator : Product  OutDataTypeStr=double
  xxeuler321_Spec_5_sin_call : Trigonometry
  xxeuler321_Spec_6_operator : Product  OutDataTypeStr=double
  xxeuler321_Spec_7_sin_call : Trigonometry
  xxeuler321_Spec_8_operator : Gain  Gain=-1  OutDataTypeStr=double
  xxeuler321_Spec_9_sin_call : Trigonometry
  valid : Outport
  wires:
  validator/1 -> valid/1
  xxeuler321_Spec_7_sin_call/1 -> xxeuler321_Spec_8_operator/1
  xxeuler321_Spec_4_cos_call/1 -> xxeuler321_Spec_6_operator/2
  xxeuler321_Spec_5_sin_call/1 -> xxeuler321_Spec_6_operator/1
  xxeuler321_Spec_50_cos_call/1 -> xxeuler321_Spec_52_operator/2
  xxeuler321_Spec_51_cos_call/1 -> xxeuler321_Spec_52_operator/1
  xxeuler321_Spec_44_operator/1 -> xxeuler321_Spec_49_operator/2
  xxeuler321_Spec_48_operator/1 -> xxeuler321_Spec_49_operator/1
  xxeuler321_Spec_45_sin_call/1 -> xxeuler321_Spec_48_operator/2
  xxeuler321_Spec_47_operator/1 -> xxeuler321_Spec_48_operator/1
  xxeuler321_Spec_46_cos_call/1 -> xxeuler321_Spec_47_operator/1
  xxeuler321_Spec_40_cos_call/1 -> xxeuler321_Spec_44_operator/2
  xxeuler321_Spec_43_operator/1 -> xxeuler321_Spec_44_operator/1
  xxeuler321_Spec_41_sin_call/1 -> xxeuler321_Spec_43_operator/2
  xxeuler321_Spec_42_sin_call/1 -> xxeuler321_Spec_43_operator/1
  xxeuler321_Spec_1_cos_call/1 -> xxeuler321_Spec_3_operator/2
  xxeuler321_Spec_2_cos_call/1 -> xxeuler321_Spec_3_operator/1
  xxeuler321_Spec_35_operator/1 -> xxeuler321_Spec_39_operator/2
  xxeuler321_Spec_38_operator/1 -> xxeuler321_Spec_39_operator/1
  xxeuler321_Spec_36_sin_call/1 -> xxeuler321_Spec_38_operator/2
  xxeuler321_Spec_37_sin_call/1 -> xxeuler321_Spec_38_operator/1
  xxeuler321_Spec_31_cos_call/1 -> xxeuler321_Spec_35_operator/2
  xxeuler321_Spec_34_operator/1 -> xxeuler321_Spec_35_operator/1
  xxeuler321_Spec_32_sin_call/1 -> xxeuler321_Spec_34_operator/2
  xxeuler321_Spec_33_cos_call/1 -> xxeuler321_Spec_34_operator/1
  xxeuler321_Spec_28_sin_call/1 -> xxeuler321_Spec_30_operator/2
  xxeuler321_Spec_29_cos_call/1 -> xxeuler321_Spec_30_operator/1
  xxeuler321_Spec_23_operator/1 -> xxeuler321_Spec_27_operator/2
  xxeuler321_Spec_26_operator/1 -> xxeuler321_Spec_27_operator/1
  xxeuler321_Spec_24_cos_call/1 -> xxeuler321_Spec_26_operator/2
  xxeuler321_Spec_25_cos_call/1 -> xxeuler321_Spec_26_operator/1
  xxeuler321_Spec_19_sin_call/1 -> xxeuler321_Spec_23_operator/2
  xxeuler321_Spec_22_operator/1 -> xxeuler321_Spec_23_operator/1
  xxeuler321_Spec_20_sin_call/1 -> xxeuler321_Spec_22_operator/2
  xxeuler321_Spec_21_sin_call/1 -> xxeuler321_Spec_22_operator/1
  xxeuler321_Spec_13_operator/1 -> xxeuler321_Spec_18_operator/2
  xxeuler321_Spec_17_operator/1 -> xxeuler321_Spec_18_operator/1
  xxeuler321_Spec_14_cos_call/1 -> xxeuler321_Spec_17_operator/2
  xxeuler321_Spec_16_operator/1 -> xxeuler321_Spec_17_operator/1
  xxeuler321_Spec_15_sin_call/1 -> xxeuler321_Spec_16_operator/1
  xxeuler321_Spec_9_sin_call/1 -> xxeuler321_Spec_13_operator/2
  xxeuler321_Spec_12_operator/1 -> xxeuler321_Spec_13_operator/1
  xxeuler321_Spec_10_sin_call/1 -> xxeuler321_Spec_12_operator/2
  xxeuler321_Spec_11_cos_call/1 -> xxeuler321_Spec_12_operator/1
  EUL001_9/1(guarantee) -> validator/9
  EUL001_8/1(guarantee) -> validator/8
  EUL001_7/1(guarantee) -> validator/7
  EUL001_6/1(guarantee) -> validator/6
  EUL001_5/1(guarantee) -> validator/5
  EUL001_4/1(guarantee) -> validator/4
  EUL001_3/1(guarantee) -> validator/3
  EUL001_2/1(guarantee) -> validator/2
  EUL001_1/1(guarantee) -> validator/1
  xxeuler321_Spec_49_operator/1 -> spec91_operator/2
  Demux3/2 -> spec91_operator/1
  xxeuler321_Spec_52_operator/1 -> spec67_operator/2
  Demux3/1 -> spec67_operator/1
  xxeuler321_Spec_3_operator/1 -> spec197_operator/2
  Demux3/9 -> spec197_operator/1
  xxeuler321_Spec_6_operator/1 -> spec187_operator/2
  Demux3/8 -> spec187_operator/1
  xxeuler321_Spec_8_operator/1 -> spec177_operator/2
  Demux3/7 -> spec177_operator/1
  xxeuler321_Spec_18_operator/1 -> spec169_operator/2
  Demux3/6 -> spec169_operator/1
  xxeuler321_Spec_27_operator/1 -> spec145_operator/2
  Demux3/5 -> spec145_operator/1
  xxeuler321_Spec_30_operator/1 -> spec123_operator/2
  Demux3/4 -> spec123_operator/1
  xxeuler321_Spec_39_operator/1 -> spec113_operator/2
  Demux3/3 -> spec113_operator/1
  spec197_operator/1 -> EUL001_9/1(In1)
  spec187_operator/1 -> EUL001_8/1(In1)
  spec177_operator/1 -> EUL001_7/1(In1)
  spec169_operator/1 -> EUL001_6/1(In1)
  spec145_operator/1 -> EUL001_5/1(In1)
  spec123_operator/1 -> EUL001_4/1(In1)
  spec113_operator/1 -> EUL001_3/1(In1)
  spec91_operator/1 -> EUL001_2/1(In1)
  spec67_operator/1 -> EUL001_1/1(In1)
  euler321_Spec_theta/1 -> xxeuler321_Spec_41_sin_call/1, xxeuler321_Spec_10_sin_call/1, xxeuler321_Spec_32_sin_call/1, xxeuler321_Spec_20_sin_call/1, xxeuler321_Spec_51_cos_call/1, xxeuler321_Spec_29_cos_call/1, xxeuler321_Spec_7_sin_call/1, xxeuler321_Spec_4_cos_call/1, xxeuler321_Spec_1_cos_call/1
  euler321_Spec_phi/1 -> xxeuler321_Spec_46_cos_call/1, xxeuler321_Spec_15_sin_call/1, xxeuler321_Spec_2_cos_call/1, xxeuler321_Spec_25_cos_call/1, xxeuler321_Spec_5_sin_call/1, xxeuler321_Spec_37_sin_call/1, xxeuler321_Spec_33_cos_call/1, xxeuler321_Spec_21_sin_call/1, xxeuler321_Spec_11_cos_call/1, xxeuler321_Spec_42_sin_call/1
  euler321_Spec_psi/1 -> xxeuler321_Spec_45_sin_call/1, xxeuler321_Spec_36_sin_call/1, xxeuler321_Spec_14_cos_call/1, xxeuler321_Spec_24_cos_call/1, xxeuler321_Spec_40_cos_call/1, xxeuler321_Spec_9_sin_call/1, xxeuler321_Spec_31_cos_call/1, xxeuler321_Spec_19_sin_call/1, xxeuler321_Spec_50_cos_call/1, xxeuler321_Spec_28_sin_call/1
  DCM321/1 -> Reshape/1
  Reshape/1 -> Demux3/1

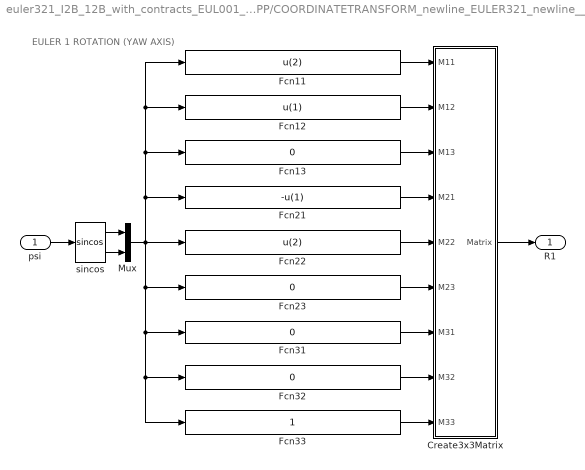
== system euler321_I2B_12B_with_contracts_EUL001_PP/COORDINATETRANSFORM_newline_EULER321_newline__lpar_INERTIALTOBODY_rpar_/Euler1Rotation_newline__lpar_Yaw_rpar_ ==
  note: EULER 1 ROTATION (YAW AXIS)
  psi : Inport
  Create3x3Matrix : Subsystem  TreatAsAtomicUnit=on  mask(Create 3x3 Matrix){}
      mask help: shared_aeroblks:sharedaeroblkutil:blockCreate3x3MatrixDesc
      mask init:
      | if license('test','aerospace_blockset')
      |     aerosharedicon('shared');
      | elseif license('test','powertrain_blockset')
      |     sharedautoicon('shared');
      | end
      mask Help: eval('if license(''test'',''aerospace_blockset'')aerosharedhelp(''create_threebythree_matrix'');elseif license(''test'',''powertrain_blockset'')sharedautohelp(''create_threebythree_matrix'');end')
      mask Display:
      | port_label('input',1,'A_{11}','texmode','on');
      | port_label('input',2,'A_{12}','texmode','on');
      | port_label('input',3,'A_{13}','texmode','on');
      | port_label('input',4,'A_{21}','texmode','on');
      | port_label('input',5,'A_{22}','texmode','on');
      | port_label('input',6,'A_{23}','texmode','on');
      | port_label('input',7,'A_{31}','texmode','on');
      | port_label('input',8,'A_{32}','texmode','on');
      | port_label('input',9,'A_{33}','texmode','on');
      | port_label('output',1,'A','texmode','on');
  Fcn11 : Fcn  Expr=u(2)
  Fcn12 : Fcn  Expr=u(1)
  Fcn{13,23,31..32} (4 alike) : Fcn  Expr=0
  Fcn21 : Fcn  Expr=-u(1)
  Fcn22 : Fcn  Expr=u(2)
  Fcn33 : Fcn  Expr=1
  Mux : Mux  Inputs=2
  sincos : Trigonometry  Operator=sincos
  R1 : Outport  PortDimensions=[3,3]  VectorParamsAs1DForOutWhenUnconnected=off
  wires:
  psi/1 -> sincos/1
  Create3x3Matrix/1(Matrix) -> R1/1
  sincos/1 -> Mux/1
  sincos/2 -> Mux/2
  Mux/1 -> Fcn32/1, Fcn33/1, Fcn31/1, Fcn23/1, Fcn22/1, Fcn11/1, Fcn12/1, Fcn13/1, Fcn21/1
  Fcn11/1 -> Create3x3Matrix/1(M11)
  Fcn12/1 -> Create3x3Matrix/2(M12)
  Fcn13/1 -> Create3x3Matrix/3(M13)
  Fcn21/1 -> Create3x3Matrix/4(M21)
  Fcn31/1 -> Create3x3Matrix/7(M31)
  Fcn22/1 -> Create3x3Matrix/5(M22)
  Fcn23/1 -> Create3x3Matrix/6(M23)
  Fcn32/1 -> Create3x3Matrix/8(M32)
  Fcn33/1 -> Create3x3Matrix/9(M33)

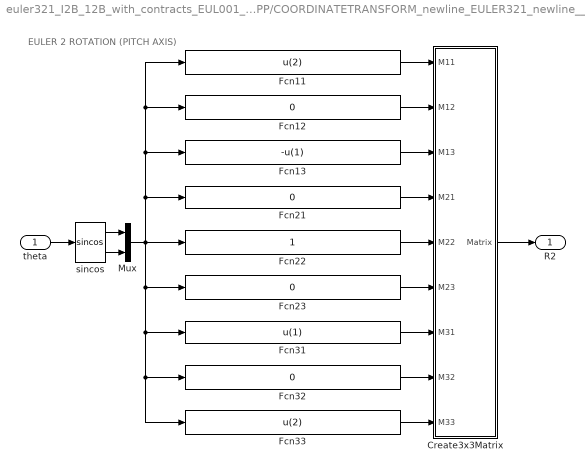
== system euler321_I2B_12B_with_contracts_EUL001_PP/COORDINATETRANSFORM_newline_EULER321_newline__lpar_INERTIALTOBODY_rpar_/Euler2Rotation_newline__lpar_Pitch_rpar_ ==
  note: EULER 2 ROTATION (PITCH AXIS)
  theta : Inport
  Create3x3Matrix : Subsystem  TreatAsAtomicUnit=on  mask(Create 3x3 Matrix){}
      mask help: shared_aeroblks:sharedaeroblkutil:blockCreate3x3MatrixDesc
      mask init:
      | if license('test','aerospace_blockset')
      |     aerosharedicon('shared');
      | elseif license('test','powertrain_blockset')
      |     sharedautoicon('shared');
      | end
      mask Help: eval('if license(''test'',''aerospace_blockset'')aerosharedhelp(''create_threebythree_matrix'');elseif license(''test'',''powertrain_blockset'')sharedautohelp(''create_threebythree_matrix'');end')
      mask Display:
      | port_label('input',1,'A_{11}','texmode','on');
      | port_label('input',2,'A_{12}','texmode','on');
      | port_label('input',3,'A_{13}','texmode','on');
      | port_label('input',4,'A_{21}','texmode','on');
      | port_label('input',5,'A_{22}','texmode','on');
      | port_label('input',6,'A_{23}','texmode','on');
      | port_label('input',7,'A_{31}','texmode','on');
      | port_label('input',8,'A_{32}','texmode','on');
      | port_label('input',9,'A_{33}','texmode','on');
      | port_label('output',1,'A','texmode','on');
  Fcn11 : Fcn  Expr=u(2)
  Fcn{12,21,23,32} (4 alike) : Fcn  Expr=0
  Fcn13 : Fcn  Expr=-u(1)
  Fcn22 : Fcn  Expr=1
  Fcn31 : Fcn  Expr=u(1)
  Fcn33 : Fcn  Expr=u(2)
  Mux : Mux  Inputs=2
  sincos : Trigonometry  Operator=sincos
  R2 : Outport  PortDimensions=[3,3]  VectorParamsAs1DForOutWhenUnconnected=off
  wires:
  theta/1 -> sincos/1
  Create3x3Matrix/1(Matrix) -> R2/1
  sincos/1 -> Mux/1
  sincos/2 -> Mux/2
  Mux/1 -> Fcn32/1, Fcn33/1, Fcn31/1, Fcn23/1, Fcn22/1, Fcn11/1, Fcn12/1, Fcn13/1, Fcn21/1
  Fcn11/1 -> Create3x3Matrix/1(M11)
  Fcn12/1 -> Create3x3Matrix/2(M12)
  Fcn13/1 -> Create3x3Matrix/3(M13)
  Fcn21/1 -> Create3x3Matrix/4(M21)
  Fcn31/1 -> Create3x3Matrix/7(M31)
  Fcn22/1 -> Create3x3Matrix/5(M22)
  Fcn23/1 -> Create3x3Matrix/6(M23)
  Fcn32/1 -> Create3x3Matrix/8(M32)
  Fcn33/1 -> Create3x3Matrix/9(M33)

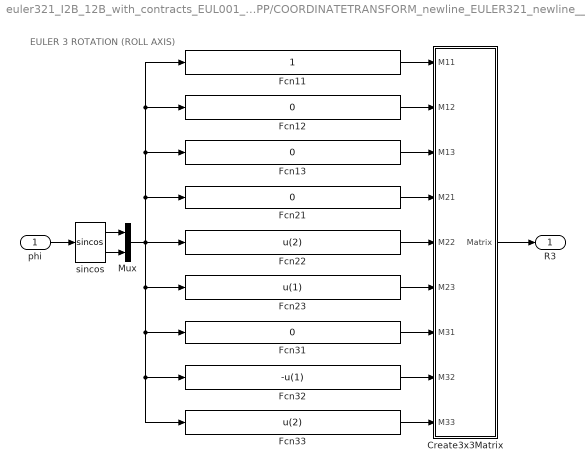
== system euler321_I2B_12B_with_contracts_EUL001_PP/COORDINATETRANSFORM_newline_EULER321_newline__lpar_INERTIALTOBODY_rpar_/Euler3Rotation_newline__lpar_Roll_rpar_ ==
  note: EULER 3 ROTATION (ROLL AXIS)
  phi : Inport
  Create3x3Matrix : Subsystem  TreatAsAtomicUnit=on  mask(Create 3x3 Matrix){}
      mask help: shared_aeroblks:sharedaeroblkutil:blockCreate3x3MatrixDesc
      mask init:
      | if license('test','aerospace_blockset')
      |     aerosharedicon('shared');
      | elseif license('test','powertrain_blockset')
      |     sharedautoicon('shared');
      | end
      mask Help: eval('if license(''test'',''aerospace_blockset'')aerosharedhelp(''create_threebythree_matrix'');elseif license(''test'',''powertrain_blockset'')sharedautohelp(''create_threebythree_matrix'');end')
      mask Display:
      | port_label('input',1,'A_{11}','texmode','on');
      | port_label('input',2,'A_{12}','texmode','on');
      | port_label('input',3,'A_{13}','texmode','on');
      | port_label('input',4,'A_{21}','texmode','on');
      | port_label('input',5,'A_{22}','texmode','on');
      | port_label('input',6,'A_{23}','texmode','on');
      | port_label('input',7,'A_{31}','texmode','on');
      | port_label('input',8,'A_{32}','texmode','on');
      | port_label('input',9,'A_{33}','texmode','on');
      | port_label('output',1,'A','texmode','on');
  Fcn11 : Fcn  Expr=1
  Fcn{12..13,21,31} (4 alike) : Fcn  Expr=0
  Fcn22 : Fcn  Expr=u(2)
  Fcn23 : Fcn  Expr=u(1)
  Fcn32 : Fcn  Expr=-u(1)
  Fcn33 : Fcn  Expr=u(2)
  Mux : Mux  Inputs=2
  sincos : Trigonometry  Operator=sincos
  R3 : Outport  PortDimensions=[3,3]  VectorParamsAs1DForOutWhenUnconnected=off
  wires:
  phi/1 -> sincos/1
  Create3x3Matrix/1(Matrix) -> R3/1
  sincos/1 -> Mux/1
  sincos/2 -> Mux/2
  Mux/1 -> Fcn32/1, Fcn33/1, Fcn31/1, Fcn23/1, Fcn22/1, Fcn11/1, Fcn12/1, Fcn13/1, Fcn21/1
  Fcn11/1 -> Create3x3Matrix/1(M11)
  Fcn12/1 -> Create3x3Matrix/2(M12)
  Fcn13/1 -> Create3x3Matrix/3(M13)
  Fcn21/1 -> Create3x3Matrix/4(M21)
  Fcn31/1 -> Create3x3Matrix/7(M31)
  Fcn22/1 -> Create3x3Matrix/5(M22)
  Fcn23/1 -> Create3x3Matrix/6(M23)
  Fcn32/1 -> Create3x3Matrix/8(M32)
  Fcn33/1 -> Create3x3Matrix/9(M33)

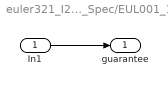
== system euler321_I2B_12B_with_contracts_EUL001_PP/euler321_I2B_12B_euler321_Spec/EUL001_1 ==
  In1 : Inport
  guarantee : Outport  OutDataTypeStr=boolean
  wires:
  In1/1 -> guarantee/1

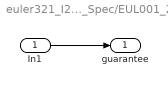
== system euler321_I2B_12B_with_contracts_EUL001_PP/euler321_I2B_12B_euler321_Spec/EUL001_2 ==
  In1 : Inport
  guarantee : Outport  OutDataTypeStr=boolean
  wires:
  In1/1 -> guarantee/1

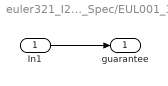
== system euler321_I2B_12B_with_contracts_EUL001_PP/euler321_I2B_12B_euler321_Spec/EUL001_3 ==
  In1 : Inport
  guarantee : Outport  OutDataTypeStr=boolean
  wires:
  In1/1 -> guarantee/1

== system euler321_I2B_12B_with_contracts_EUL001_PP/euler321_I2B_12B_euler321_Spec/EUL001_4 ==
  In1 : Inport
  guarantee : Outport  OutDataTypeStr=boolean
  wires:
  In1/1 -> guarantee/1

== system euler321_I2B_12B_with_contracts_EUL001_PP/euler321_I2B_12B_euler321_Spec/EUL001_5 ==
  In1 : Inport
  guarantee : Outport  OutDataTypeStr=boolean
  wires:
  In1/1 -> guarantee/1

== system euler321_I2B_12B_with_contracts_EUL001_PP/euler321_I2B_12B_euler321_Spec/EUL001_6 ==
  In1 : Inport
  guarantee : Outport  OutDataTypeStr=boolean
  wires:
  In1/1 -> guarantee/1

== system euler321_I2B_12B_with_contracts_EUL001_PP/euler321_I2B_12B_euler321_Spec/EUL001_7 ==
  In1 : Inport
  guarantee : Outport  OutDataTypeStr=boolean
  wires:
  In1/1 -> guarantee/1

== system euler321_I2B_12B_with_contracts_EUL001_PP/euler321_I2B_12B_euler321_Spec/EUL001_8 ==
  In1 : Inport
  guarantee : Outport  OutDataTypeStr=boolean
  wires:
  In1/1 -> guarantee/1

== system euler321_I2B_12B_with_contracts_EUL001_PP/euler321_I2B_12B_euler321_Spec/EUL001_9 ==
  In1 : Inport
  guarantee : Outport  OutDataTypeStr=boolean
  wires:
  In1/1 -> guarantee/1

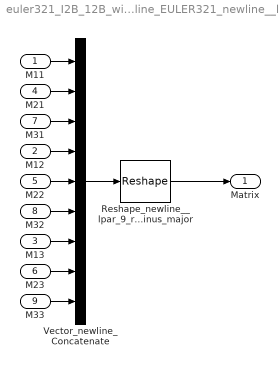
== system euler321_I2B_12B_with_contracts_EUL001_PP/COORDINATETRANSFORM_newline_EULER321_newline__lpar_INERTIALTOBODY_rpar_/Euler1Rotation_newline__lpar_Yaw_rpar_/Create3x3Matrix ==
  M11 : Inport  PortDimensions=1
  M12 : Inport  Port=2  PortDimensions=1
  M13 : Inport  Port=3  PortDimensions=1
  M21 : Inport  Port=4  PortDimensions=1
  M22 : Inport  Port=5  PortDimensions=1
  M23 : Inport  Port=6  PortDimensions=1
  M31 : Inport  Port=7  PortDimensions=1
  M32 : Inport  Port=8  PortDimensions=1
  M33 : Inport  Port=9  PortDimensions=1
  Reshape_newline__lpar_9_rpar_to_lsbrak_3x3_rsbrak__newline_column_minus_major : Reshape  OutputDimensionality=Customize  OutputDimensions=[3,3]
  Vector_newline_Concatenate : Concatenate  NumInputs=9
  Matrix : Outport  PortDimensions=[3 3]  VectorParamsAs1DForOutWhenUnconnected=off
  wires:
  M33/1 -> Vector_newline_Concatenate/9
  M23/1 -> Vector_newline_Concatenate/8
  M13/1 -> Vector_newline_Concatenate/7
  M32/1 -> Vector_newline_Concatenate/6
  Reshape_newline__lpar_9_rpar_to_lsbrak_3x3_rsbrak__newline_column_minus_major/1 -> Matrix/1
  M22/1 -> Vector_newline_Concatenate/5
  M12/1 -> Vector_newline_Concatenate/4
  M31/1 -> Vector_newline_Concatenate/3
  M21/1 -> Vector_newline_Concatenate/2
  M11/1 -> Vector_newline_Concatenate/1
  Vector_newline_Concatenate/1 -> Reshape_newline__lpar_9_rpar_to_lsbrak_3x3_rsbrak__newline_column_minus_major/1

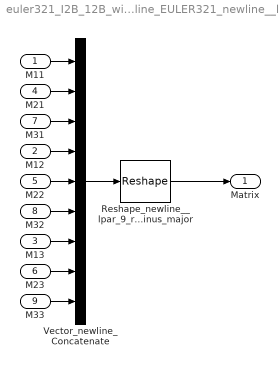
== system euler321_I2B_12B_with_contracts_EUL001_PP/COORDINATETRANSFORM_newline_EULER321_newline__lpar_INERTIALTOBODY_rpar_/Euler2Rotation_newline__lpar_Pitch_rpar_/Create3x3Matrix ==
  M11 : Inport  PortDimensions=1
  M12 : Inport  Port=2  PortDimensions=1
  M13 : Inport  Port=3  PortDimensions=1
  M21 : Inport  Port=4  PortDimensions=1
  M22 : Inport  Port=5  PortDimensions=1
  M23 : Inport  Port=6  PortDimensions=1
  M31 : Inport  Port=7  PortDimensions=1
  M32 : Inport  Port=8  PortDimensions=1
  M33 : Inport  Port=9  PortDimensions=1
  Reshape_newline__lpar_9_rpar_to_lsbrak_3x3_rsbrak__newline_column_minus_major : Reshape  OutputDimensionality=Customize  OutputDimensions=[3,3]
  Vector_newline_Concatenate : Concatenate  NumInputs=9
  Matrix : Outport  PortDimensions=[3 3]  VectorParamsAs1DForOutWhenUnconnected=off
  wires:
  M33/1 -> Vector_newline_Concatenate/9
  M23/1 -> Vector_newline_Concatenate/8
  M13/1 -> Vector_newline_Concatenate/7
  M32/1 -> Vector_newline_Concatenate/6
  Reshape_newline__lpar_9_rpar_to_lsbrak_3x3_rsbrak__newline_column_minus_major/1 -> Matrix/1
  M22/1 -> Vector_newline_Concatenate/5
  M12/1 -> Vector_newline_Concatenate/4
  M31/1 -> Vector_newline_Concatenate/3
  M21/1 -> Vector_newline_Concatenate/2
  M11/1 -> Vector_newline_Concatenate/1
  Vector_newline_Concatenate/1 -> Reshape_newline__lpar_9_rpar_to_lsbrak_3x3_rsbrak__newline_column_minus_major/1

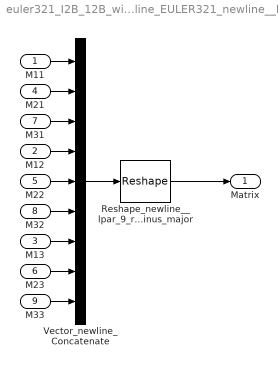
== system euler321_I2B_12B_with_contracts_EUL001_PP/COORDINATETRANSFORM_newline_EULER321_newline__lpar_INERTIALTOBODY_rpar_/Euler3Rotation_newline__lpar_Roll_rpar_/Create3x3Matrix ==
  M11 : Inport  PortDimensions=1
  M12 : Inport  Port=2  PortDimensions=1
  M13 : Inport  Port=3  PortDimensions=1
  M21 : Inport  Port=4  PortDimensions=1
  M22 : Inport  Port=5  PortDimensions=1
  M23 : Inport  Port=6  PortDimensions=1
  M31 : Inport  Port=7  PortDimensions=1
  M32 : Inport  Port=8  PortDimensions=1
  M33 : Inport  Port=9  PortDimensions=1
  Reshape_newline__lpar_9_rpar_to_lsbrak_3x3_rsbrak__newline_column_minus_major : Reshape  OutputDimensionality=Customize  OutputDimensions=[3,3]
  Vector_newline_Concatenate : Concatenate  NumInputs=9
  Matrix : Outport  PortDimensions=[3 3]  VectorParamsAs1DForOutWhenUnconnected=off
  wires:
  M33/1 -> Vector_newline_Concatenate/9
  M23/1 -> Vector_newline_Concatenate/8
  M13/1 -> Vector_newline_Concatenate/7
  M32/1 -> Vector_newline_Concatenate/6
  Reshape_newline__lpar_9_rpar_to_lsbrak_3x3_rsbrak__newline_column_minus_major/1 -> Matrix/1
  M22/1 -> Vector_newline_Concatenate/5
  M12/1 -> Vector_newline_Concatenate/4
  M31/1 -> Vector_newline_Concatenate/3
  M21/1 -> Vector_newline_Concatenate/2
  M11/1 -> Vector_newline_Concatenate/1
  Vector_newline_Concatenate/1 -> Reshape_newline__lpar_9_rpar_to_lsbrak_3x3_rsbrak__newline_column_minus_major/1
